simulink model "simulink_tp2"  (R2025b)
settings: Solver=VariableStepAuto  StartTime=0.0  StopTime=600  RelTol=1e-3
values from neighbouring files (symbols this model uses):
  f = 7.2 * 10^-5    (= 7.2e-05)    [script_tp1.m]    (also in script_tp2.m = 0.0019)
  J = 1.29 * 10^-4    (= 0.000129)    [script_tp1.m]    (also in script_tp2.m = 0.411)
  K = Kem / (R * f + Kem^2)    (= 9.89738392348)    [script_tp1.m]    (also in script_tp2.m)
  Ke = 1.1    [script_tp2.m]
  Kf = 1.007    [script_tp2.m]
  Kh = 2.170    (= 2.17)    [script_tp2.m]
  Kp = 10    [script_tp1.m]    (also in script_tp2.m = 100)
  Kw = 10 / 3000    (= 0.00333333333333)    [script_tp1.m]    (also in script_tp2.m)
  L = 5.610 * 10^-4    (= 0.000561)    [script_tp1.m]    (also in script_tp2.m = 83.9)
  Ra = 3.58    [script_tp2.m]
  Tel = L / R    (= 0.000389583333333)    [script_tp1.m]    (also in script_tp2.m)
  Tem = (R*J)/ (R*f + Kem ^ 2)    (= 0.0183853803763)    [script_tp1.m]    (also in script_tp2.m)
libraries: simulink x1, slpidlib x1
settings Model: Creator=Ahmed  LastModifiedBy=Ahmed

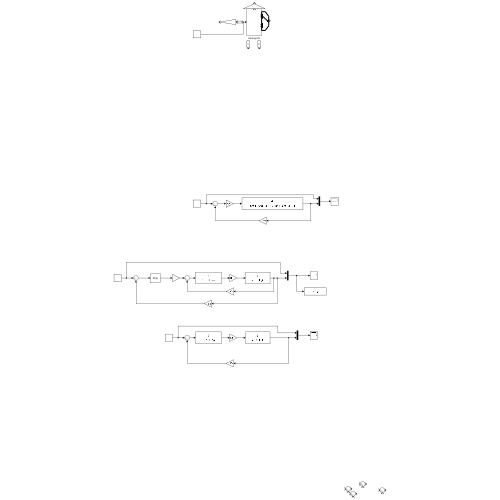
[thumbnail: Simulink's stored preview of the top-level diagram]
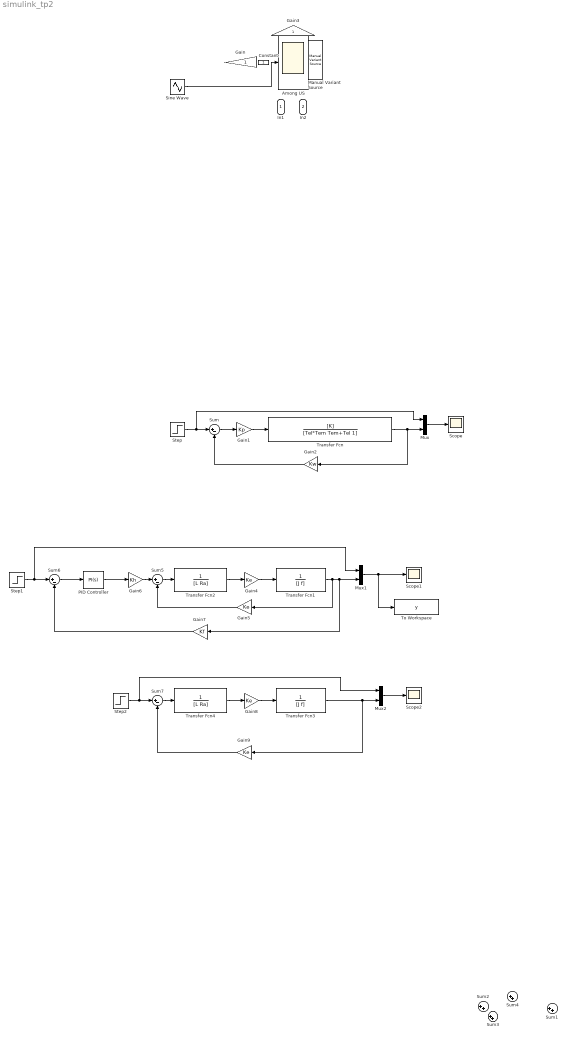
== system simulink_tp2 ==
  In1 : Inport
  In2 : Inport  Port=2
  Among US : Scope
      settings: ActiveDisplayYMinimum=-1  ActiveDisplayYMaximum=1
  Constant : Constant
  Gain : Gain
  Gain1 : Gain  Gain=Kp
  Gain2 : Gain  Gain=Kw
  Gain3 : Gain
  Gain{4..5,8..9} (4 alike) : Gain  Gain=Ke
  Gain6 : Gain  Gain=Kh
  Gain7 : Gain  Gain=Kf
  Manual Variant Source : simulink/Signal Routing/Manual Variant Source  NumChoices=2  LabelModeActiveChoice=V_1
  Mux : Mux  Inputs=2
  Mux1 : Mux  Inputs=2
  Mux2 : Mux  Inputs=2
  PID Controller : slpidlib/PID Controller  Controller=PI  Form=Parallel  TimeDomain=Continuous-time  UseExternalTs=off  SampleTime=-1  IntegratorMethod=Forward Euler  FilterMethod=Forward Euler  ControllerParametersSource=internal  P=0.005  I=1/100  UseKiTs=off  D=0  UseExternalDerivativeSource=off  N=100  UseFilter=on  TunerSelectOption=Transfer Function Based (PID Tuner App)  InitialConditionSource=internal  InitialConditionForIntegrator=0  InitialConditionForFilter=0  DifferentiatorICPrevScaledInput=0  ExternalReset=none  TrackingMode=off  Kt=1  LimitOutput=off  SatLimitsSource=internal  UpperSaturationLimit=inf  LowerSaturationLimit=-inf  LinearizeAsGain=on  AntiWindupMode=none  Kb=1  LimitIntegrator=off  UpperIntegratorSaturationLimit=inf  LowerIntegratorSaturationLimit=-inf  POutMin=[]  POutMax=[]  IOutMin=[]  IOutMax=[]  DOutMin=[]  DOutMax=[]  NOutMin=[]  NOutMax=[]  SumOutMin=[]  SumOutMax=[]  SaturationOutMin=[]  SaturationOutMax=[]  PParamMin=[]  PParamMax=[]  IParamMin=[]  IParamMax=[]  DParamMin=[]  DParamMax=[]  NParamMin=[]  NParamMax=[]  KbParamMin=[]  KbParamMax=[]  KtParamMin=[]  KtParamMax=[]  KbOutMin=[]  KbOutMax=[]  KtOutMin=[]  KtOutMax=[]  IntegratorOutMin=[]  IntegratorOutMax=[]  FilterOutMin=[]  FilterOutMax=[]  SumI1OutMin=[]  SumI1OutMax=[]  SumI2OutMin=[]  SumI2OutMax=[]  SumI3OutMin=[]  SumI3OutMax=[]  SumI4OutMin=[]  SumI4OutMax=[]  SumDOutMin=[]  SumDOutMax=[]  DifferentiatorOutMin=[]  DifferentiatorOutMax=[]  FilterDiffOutCoefMin=[]  FilterDiffOutCoefMax=[]  ReciprocalOutMin=[]  ReciprocalOutMax=[]  SumDenOutMin=[]  SumDenOutMax=[]  SumNumOutMin=[]  SumNumOutMax=[]  DivideOutMin=[]  DivideOutMax=[]  UdiffTsProdOutMin=[]  UdiffTsProdOutMax=[]  NTsProdOutMin=[]  NTsProdOutMax=[]  UintegralTsProdOutMin=[]  UintegralTsProdOutMax=[]  UngainTsProdOutMin=[]  UngainTsProdOutMax=[]  ClampingZeroOutDataTypeStr=Inherit: Inherit via back propagation  ClampingZeroOutMin=[]  ClampingZeroOutMax=[]  FilterDenConstantOutDataTypeStr=Inherit: Inherit via back propagation  FilterDenConstantOutMin=[]  FilterDenConstantOutMax=[]  PCopyOutDataTypeStr=Inherit: Inherit via back propagation  PCopyOutMin=[]  PCopyOutMax=[]  NCopyOutDataTypeStr=Inherit: Inherit via back propagation  NCopyOutMin=[]  NCopyOutMax=[]  IntegratorContinuousStateAttributes=''  IntegratorStateMustResolveToSignalObject=off  IntegratorRTWStateStorageClass=Auto  FilterContinuousStateAttributes=''  FilterStateMustResolveToSignalObject=off  FilterRTWStateStorageClass=Auto  ParallelPVariant=InternalParameters  IdealPVariant=Disabled  IVariant=InternalParameters  DVariant=Disabled  IntegratorVariant=Continuous  SatVariant=Disabled  AWVariant=Passthrough  PCopyVariant=Disabled  TRVariant=Disabled  FdbkBlocksVariant=Forward  IdealPFdbkVariant=Disabled  SatFdbkVariant=Disabled  DerivativeFilterVariant=Disabled  NVariant=Disabled  NCopyVariant=Disabled_SignalSpec  FilterICVariant=Disabled  IntegratorICVariant=InternalICs  ExternalResetVariant=Disabled  TRSumVariant=Passthrough  SumFdbkVariant=Disabled  SumVariant=Sum_PI  TsampFilterVariant=InternalTs  TsampNgainVariant=Passthrough  TsampIntegralVariant=Disabled_SignalSpec  ExternalSaturationOutDataTypeStr=Inherit: Same as second input  DerivativeSourceVariant=Disabled  PreIntVariant=InternalPreInt
  Scope : Scope
      settings: ActiveDisplayYMinimum=-1  ActiveDisplayYMaximum=1
  Scope1 : Scope
      settings: ActiveDisplayYMinimum=-1.1874999999999998  ActiveDisplayYMaximum=10.6875  DataLoggingVariableName=ScopeData2
  Scope2 : Scope
      settings: ActiveDisplayYMinimum=-6.1803050798466757  ActiveDisplayYMaximum=15.616638489104915  DataLoggingVariableName=ScopeData3
  Sine Wave : Sin  Amplitude=1.5  SampleTime=0
  Step : Step  Time=0  SampleTime=0
  Step1 : Step  Time=0  After=9.5  SampleTime=0
  Step2 : Step  Time=0  After=9.5  SampleTime=0
  Sum{,5..7} (4 alike) : Sum  Inputs=|+-
  Sum{1..4} (4 alike) : Sum  Inputs=|++
  To Workspace : ToWorkspace  VariableName=y  SampleTime=-1
      settings: Save2DSignal=2-D array (concatenate along first dimension)
  Transfer Fcn : TransferFcn  Numerator=[K]  Denominator=[Tel*Tem Tem+Tel 1]
  Transfer Fcn1 : TransferFcn  Denominator=[J f]
  Transfer Fcn2 : TransferFcn  Denominator=[L Ra]
  Transfer Fcn3 : TransferFcn  Denominator=[J f]
  Transfer Fcn4 : TransferFcn  Denominator=[L Ra]
  wires:
  Sine Wave/1 -> Among US/1
  Sum/1 -> Gain1/1
  Gain1/1 -> Transfer Fcn/1
  Gain2/1 -> Sum/2
  Transfer Fcn/1 -> Mux/2, Gain2/1
  Step/1 -> Mux/1, Sum/1
  Mux/1 -> Scope/1
  Gain5/1 -> Sum5/2
  Sum5/1 -> Transfer Fcn2/1
  Transfer Fcn2/1 -> Gain4/1
  Gain4/1 -> Transfer Fcn1/1
  Gain6/1 -> Sum5/1
  Gain7/1 -> Sum6/2
  Gain8/1 -> Transfer Fcn3/1
  Gain9/1 -> Sum7/2
  Transfer Fcn3/1 -> Mux2/2, Gain9/1
  Transfer Fcn4/1 -> Gain8/1
  Sum7/1 -> Transfer Fcn4/1
  Step2/1 -> Mux2/1, Sum7/1
  Mux2/1 -> Scope2/1
  Transfer Fcn1/1 -> Mux1/2, Gain7/1, Gain5/1
  Step1/1 -> Mux1/1, Sum6/1
  Mux1/1 -> Scope1/1, To Workspace/1
  Sum6/1 -> PID Controller/1
  PID Controller/1 -> Gain6/1
